simulink model "Q3_4706"  (R2015a)
settings: Solver=ode45  StartTime=0.0  StopTime=0.0000001  RelTol=1e-3
values from neighbouring files (symbols this model uses):
  a = gm/(cp)    (= 442336245625)    [dan_Q3_CTLE.m]
  b = (1+(gm*rs/2))/(rs*cs)    (= 31415915302.7)    [dan_Q3_CTLE.m]
  c = 1/(rd*cp)    (= 62831853071.8)    [dan_Q3_CTLE.m]
  d = 1/(rs*cs)    (= 6283183060.54)    [dan_Q3_CTLE.m]
settings Model: Creator=Danilo Vucetic  LastModifiedBy=Danilo Vucetic

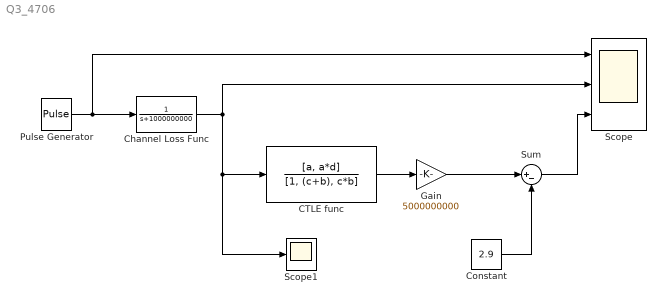
== system Q3_4706 ==
  CTLE func : TransferFcn  Numerator=[a, a*d]  Denominator=[1, (c+b), c*b]
  Channel Loss Func : TransferFcn  Denominator=[1 1000000000]
  Constant : Constant  Value=2.9
  Gain : Gain  Gain=5000000000
  Pulse Generator : DiscretePulseGenerator  PulseType=Time based  Period=0.0000000001  PulseWidth=50
  Scope : Scope  NumInputPorts=3
      settings: YMin=0~-5~-5  YMax=550000~5~5
  Scope1 : Scope
  Sum : Sum  Inputs=|+-
  wires:
  Pulse Generator/1 -> Scope/1, Channel Loss Func/1
  Channel Loss Func/1 -> Scope1/1, CTLE func/1, Scope/2
  Gain/1 -> Sum/1
  Sum/1 -> Scope/3
  Constant/1 -> Sum/2
  CTLE func/1 -> Gain/1
